simulink model "Functional_LineFollowingRobot"  (R2024a)
settings: Solver=VariableStepAuto  StartTime=0.0  StopTime=10.0  RelTol=1e-3
settings Model: Creator=pedro  LastModifiedBy=pedro

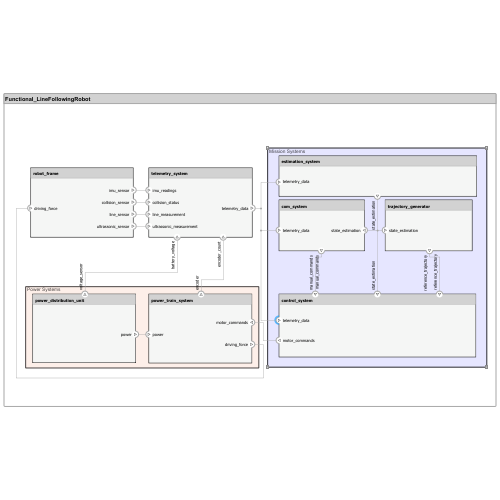
[thumbnail: Simulink's stored preview of the top-level diagram]
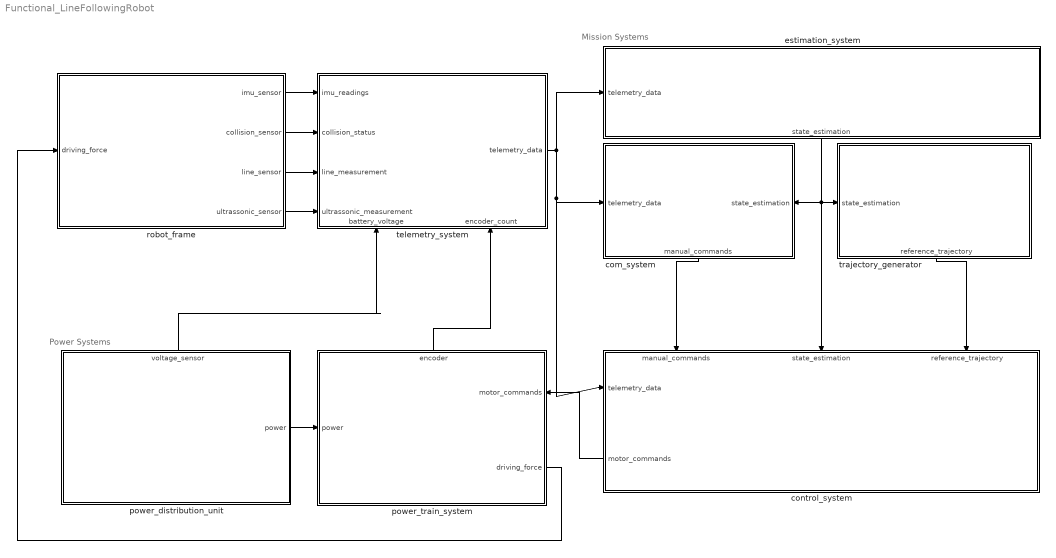
== system Functional_LineFollowingRobot ==
  note: Power Systems
  note: Mission Systems
  com_system : Subsystem
      settings: PortSchema="{\"entries\":[{\"content\":{\"headerSize\":26,\"margin\":15,\"minimumSpacing\":25,\"sides\":[{\"content\":{\"connectorIds\":[\"In2\"]},\"type\":\"ConnectorPlacement.EquallySpacedRectSide\",\"uuid\":\"4832beee-3c8d-4276-aac4-b86a684a787e\"},{\"content\":{\"connectorIds\":[\"In1\"],\"side\":\"RIGHT\"},\"type\":\"ConnectorPlacement.EquallySpacedRectSide\",\"uuid\":\"2c389b1c-5dd0-4d5d-98eb-a9eff98bcfdd\"},{\"content\":{\"side\":\"TOP\"},\"type\":\"ConnectorPlacement.EquallySpacedRectSide\",\"uuid\":\"c0c925d2-d939-46f6-a0f7-d4e3ec744eed\"},{\"content\":{\"connectorIds\":[\"Out1\"],\"side\":\"BOTTOM\"},\"type\":\"ConnectorPlacement.EquallySpacedRectSide\",\"uuid\":\"501e751b-5f5c-4d33-aa26-8cd64b6f3e74\"}]},\"type\":\"ConnectorPlacement.EquallySpacedConnector\",\"uuid\":\"424459fb-a04f-4037-ace5-d153f52e2b89\"}],\"packageUris\":[\"http://schema.mathworks.com/mf0/Connector/R2020b\"],\"version\":\"1.0\"}"
  control_system : Subsystem
      settings: PortSchema="{\"entries\":[{\"content\":{\"headerSize\":26,\"margin\":15,\"minimumSpacing\":25,\"sides\":[{\"content\":{\"connectorIds\":[\"In2\",\"Out1\"]},\"type\":\"ConnectorPlacement.EquallySpacedRectSide\",\"uuid\":\"4832beee-3c8d-4276-aac4-b86a684a787e\"},{\"content\":{\"side\":\"RIGHT\"},\"type\":\"ConnectorPlacement.EquallySpacedRectSide\",\"uuid\":\"2c389b1c-5dd0-4d5d-98eb-a9eff98bcfdd\"},{\"content\":{\"connectorIds\":[\"In1\",\"In4\",\"In3\"],\"side\":\"TOP\"},\"type\":\"ConnectorPlacement.EquallySpacedRectSide\",\"uuid\":\"c0c925d2-d939-46f6-a0f7-d4e3ec744eed\"},{\"content\":{\"side\":\"BOTTOM\"},\"type\":\"ConnectorPlacement.EquallySpacedRectSide\",\"uuid\":\"08be73b3-c42a-4f82-a3e3-56e96afeafa7\"}]},\"type\":\"ConnectorPlacement.EquallySpacedConnector\",\"uuid\":\"424459fb-a04f-4037-ace5-d153f52e2b89\"}],\"packageUris\":[\"http://schema.mathworks.com/mf0/Connector/R2020b\"],\"version\":\"1.0\"}"
  estimation_system : Subsystem
      settings: PortSchema="{\"entries\":[{\"content\":{\"headerSize\":26,\"margin\":15,\"minimumSpacing\":25,\"sides\":[{\"content\":{\"connectorIds\":[\"In1\"]},\"type\":\"ConnectorPlacement.EquallySpacedRectSide\",\"uuid\":\"4832beee-3c8d-4276-aac4-b86a684a787e\"},{\"content\":{\"side\":\"RIGHT\"},\"type\":\"ConnectorPlacement.EquallySpacedRectSide\",\"uuid\":\"2c389b1c-5dd0-4d5d-98eb-a9eff98bcfdd\"},{\"content\":{\"side\":\"TOP\"},\"type\":\"ConnectorPlacement.EquallySpacedRectSide\",\"uuid\":\"c0c925d2-d939-46f6-a0f7-d4e3ec744eed\"},{\"content\":{\"connectorIds\":[\"Out1\"],\"side\":\"BOTTOM\"},\"type\":\"ConnectorPlacement.EquallySpacedRectSide\",\"uuid\":\"d76891fa-23de-4411-a90a-4a1fbb70c268\"}]},\"type\":\"ConnectorPlacement.EquallySpacedConnector\",\"uuid\":\"424459fb-a04f-4037-ace5-d153f52e2b89\"}],\"packageUris\":[\"http://schema.mathworks.com/mf0/Connector/R2020b\"],\"version\":\"1.0\"}"
  power_distribution_unit : Subsystem
      settings: PortSchema="{\"entries\":[{\"content\":{\"headerSize\":26,\"margin\":15,\"minimumSpacing\":25,\"sides\":[{\"content\":{},\"type\":\"ConnectorPlacement.EquallySpacedRectSide\",\"uuid\":\"4832beee-3c8d-4276-aac4-b86a684a787e\"},{\"content\":{\"connectorIds\":[\"Out1\"],\"side\":\"RIGHT\"},\"type\":\"ConnectorPlacement.EquallySpacedRectSide\",\"uuid\":\"2c389b1c-5dd0-4d5d-98eb-a9eff98bcfdd\"},{\"content\":{\"connectorIds\":[\"Out2\"],\"side\":\"TOP\"},\"type\":\"ConnectorPlacement.EquallySpacedRectSide\",\"uuid\":\"c0c925d2-d939-46f6-a0f7-d4e3ec744eed\"},{\"content\":{\"side\":\"BOTTOM\"},\"type\":\"ConnectorPlacement.EquallySpacedRectSide\",\"uuid\":\"1aa9b233-1b30-4eb2-b648-626ea5c748e2\"}]},\"type\":\"ConnectorPlacement.EquallySpacedConnector\",\"uuid\":\"424459fb-a04f-4037-ace5-d153f52e2b89\"}],\"packageUris\":[\"http://schema.mathworks.com/mf0/Connector/R2020b\"],\"version\":\"1.0\"}"
  power_train_system : Subsystem
      settings: PortSchema="{\"entries\":[{\"content\":{\"headerSize\":26,\"margin\":15,\"minimumSpacing\":25,\"sides\":[{\"content\":{\"connectorIds\":[\"In2\"]},\"type\":\"ConnectorPlacement.EquallySpacedRectSide\",\"uuid\":\"4832beee-3c8d-4276-aac4-b86a684a787e\"},{\"content\":{\"connectorIds\":[\"In1\",\"Out1\"],\"side\":\"RIGHT\"},\"type\":\"ConnectorPlacement.EquallySpacedRectSide\",\"uuid\":\"2c389b1c-5dd0-4d5d-98eb-a9eff98bcfdd\"},{\"content\":{\"connectorIds\":[\"Out2\"],\"side\":\"TOP\"},\"type\":\"ConnectorPlacement.EquallySpacedRectSide\",\"uuid\":\"c0c925d2-d939-46f6-a0f7-d4e3ec744eed\"},{\"content\":{\"side\":\"BOTTOM\"},\"type\":\"ConnectorPlacement.EquallySpacedRectSide\",\"uuid\":\"cbeccc70-c914-499a-a0c2-ba0cf3f08829\"}]},\"type\":\"ConnectorPlacement.EquallySpacedConnector\",\"uuid\":\"424459fb-a04f-4037-ace5-d153f52e2b89\"}],\"packageUris\":[\"http://schema.mathworks.com/mf0/Connector/R2020b\"],\"version\":\"1.0\"}"
  robot_frame : Subsystem
      settings: PortSchema="{\"entries\":[{\"content\":{\"headerSize\":26,\"margin\":15,\"minimumSpacing\":25,\"sides\":[{\"content\":{\"connectorIds\":[\"In1\"]},\"type\":\"ConnectorPlacement.EquallySpacedRectSide\",\"uuid\":\"4832beee-3c8d-4276-aac4-b86a684a787e\"},{\"content\":{\"connectorIds\":[\"Out1\",\"Out2\",\"Out3\",\"Out4\"],\"side\":\"RIGHT\"},\"type\":\"ConnectorPlacement.EquallySpacedRectSide\",\"uuid\":\"2c389b1c-5dd0-4d5d-98eb-a9eff98bcfdd\"},{\"content\":{\"side\":\"TOP\"},\"type\":\"ConnectorPlacement.EquallySpacedRectSide\",\"uuid\":\"c0c925d2-d939-46f6-a0f7-d4e3ec744eed\"}]},\"type\":\"ConnectorPlacement.EquallySpacedConnector\",\"uuid\":\"424459fb-a04f-4037-ace5-d153f52e2b89\"}],\"packageUris\":[\"http://schema.mathworks.com/mf0/Connector/R2020b\"],\"version\":\"1.0\"}"
  telemetry_system : Subsystem
      settings: PortSchema="{\"entries\":[{\"content\":{\"headerSize\":26,\"margin\":15,\"minimumSpacing\":25,\"sides\":[{\"content\":{\"connectorIds\":[\"In1\",\"In2\",\"In3\",\"In4\"]},\"type\":\"ConnectorPlacement.EquallySpacedRectSide\",\"uuid\":\"4832beee-3c8d-4276-aac4-b86a684a787e\"},{\"content\":{\"connectorIds\":[\"Out1\"],\"side\":\"RIGHT\"},\"type\":\"ConnectorPlacement.EquallySpacedRectSide\",\"uuid\":\"2c389b1c-5dd0-4d5d-98eb-a9eff98bcfdd\"},{\"content\":{\"side\":\"TOP\"},\"type\":\"ConnectorPlacement.EquallySpacedRectSide\",\"uuid\":\"c0c925d2-d939-46f6-a0f7-d4e3ec744eed\"},{\"content\":{\"connectorIds\":[\"In5\",\"In6\"],\"side\":\"BOTTOM\"},\"type\":\"ConnectorPlacement.EquallySpacedRectSide\",\"uuid\":\"5c99a527-2db7-49a5-9f4f-18d6a8edb429\"}]},\"type\":\"ConnectorPlacement.EquallySpacedConnector\",\"uuid\":\"424459fb-a04f-4037-ace5-d153f52e2b89\"}],\"packageUris\":[\"http://schema.mathworks.com/mf0/Connector/R2020b\"],\"version\":\"1.0\"}"
  trajectory_generator : Subsystem
      settings: PortSchema="{\"entries\":[{\"content\":{\"headerSize\":26,\"margin\":15,\"minimumSpacing\":25,\"sides\":[{\"content\":{\"connectorIds\":[\"In1\"]},\"type\":\"ConnectorPlacement.EquallySpacedRectSide\",\"uuid\":\"4832beee-3c8d-4276-aac4-b86a684a787e\"},{\"content\":{\"side\":\"RIGHT\"},\"type\":\"ConnectorPlacement.EquallySpacedRectSide\",\"uuid\":\"2c389b1c-5dd0-4d5d-98eb-a9eff98bcfdd\"},{\"content\":{\"side\":\"TOP\"},\"type\":\"ConnectorPlacement.EquallySpacedRectSide\",\"uuid\":\"c0c925d2-d939-46f6-a0f7-d4e3ec744eed\"},{\"content\":{\"connectorIds\":[\"Out1\"],\"side\":\"BOTTOM\"},\"type\":\"ConnectorPlacement.EquallySpacedRectSide\",\"uuid\":\"37185e83-8287-462f-8b6c-e2b7cde56f21\"}]},\"type\":\"ConnectorPlacement.EquallySpacedConnector\",\"uuid\":\"424459fb-a04f-4037-ace5-d153f52e2b89\"}],\"packageUris\":[\"http://schema.mathworks.com/mf0/Connector/R2020b\"],\"version\":\"1.0\"}"
  wires:
  power_train_system/2(encoder) -> telemetry_system/6(encoder_count)
  power_distribution_unit/2(voltage_sensor) -> telemetry_system/5(battery_voltage)
  robot_frame/4(ultrassonic_sensor) -> telemetry_system/4(ultrassonic_measurement)
  robot_frame/3(line_sensor) -> telemetry_system/3(line_measurement)
  robot_frame/2(collision_sensor) -> telemetry_system/2(collision_status)
  telemetry_system/1(telemetry_data) -> control_system/2(telemetry_data), com_system/2(telemetry_data), estimation_system/1(telemetry_data)
  robot_frame/1(imu_sensor) -> telemetry_system/1(imu_readings)
  estimation_system/1(state_estimation) -> control_system/4(state_estimation), com_system/1(state_estimation), trajectory_generator/1(state_estimation)
  power_distribution_unit/1(power) -> power_train_system/2(power)
  control_system/1(motor_commands) -> power_train_system/1(motor_commands)
  com_system/1(manual_commands) -> control_system/1(manual_commands)
  trajectory_generator/1(reference_trajectory) -> control_system/3(reference_trajectory)
  power_train_system/1(driving_force) -> robot_frame/1(driving_force)

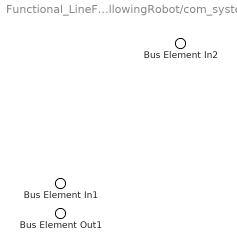
== system Functional_LineFollowingRobot/com_system ==
  Bus Element In2 : Inport  PortName=state_estimation
  Bus Element In1 : Inport  Port=2  PortName=telemetry_data
  Bus Element Out1 : Outport  PortName=manual_commands

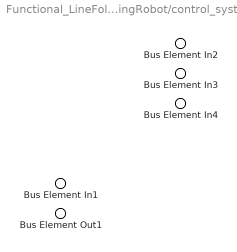
== system Functional_LineFollowingRobot/control_system ==
  Bus Element In3 : Inport  PortName=manual_commands
  Bus Element In2 : Inport  Port=2  PortName=telemetry_data
  Bus Element In4 : Inport  Port=3  PortName=reference_trajectory
  Bus Element In1 : Inport  Port=4  PortName=state_estimation
  Bus Element Out1 : Outport  PortName=motor_commands

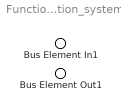
== system Functional_LineFollowingRobot/estimation_system ==
  Bus Element In1 : Inport  PortName=telemetry_data
  Bus Element Out1 : Outport  PortName=state_estimation

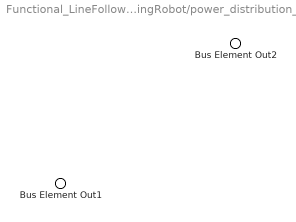
== system Functional_LineFollowingRobot/power_distribution_unit ==
  Bus Element Out2 : Outport  PortName=power
  Bus Element Out1 : Outport  Port=2  PortName=voltage_sensor

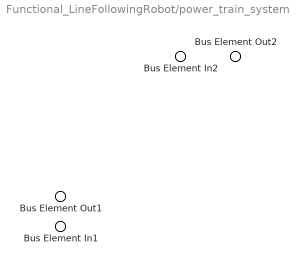
== system Functional_LineFollowingRobot/power_train_system ==
  Bus Element In2 : Inport  PortName=motor_commands
  Bus Element In1 : Inport  Port=2  PortName=power
  Bus Element Out2 : Outport  PortName=driving_force
  Bus Element Out1 : Outport  Port=2  PortName=encoder

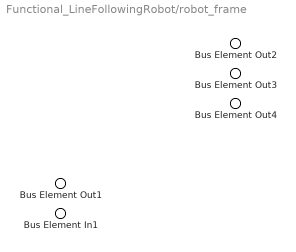
== system Functional_LineFollowingRobot/robot_frame ==
  Bus Element In1 : Inport  PortName=driving_force
  Bus Element Out4 : Outport  PortName=imu_sensor
  Bus Element Out3 : Outport  Port=2  PortName=collision_sensor
  Bus Element Out2 : Outport  Port=3  PortName=line_sensor
  Bus Element Out1 : Outport  Port=4  PortName=ultrassonic_sensor

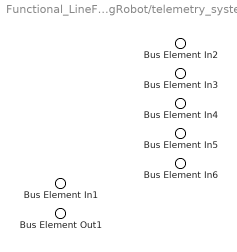
== system Functional_LineFollowingRobot/telemetry_system ==
  Bus Element In6 : Inport  PortName=imu_readings
  Bus Element In5 : Inport  Port=2  PortName=collision_status
  Bus Element In4 : Inport  Port=3  PortName=line_measurement
  Bus Element In3 : Inport  Port=4  PortName=ultrassonic_measurement
  Bus Element In2 : Inport  Port=5  PortName=battery_voltage
  Bus Element In1 : Inport  Port=6  PortName=encoder_count
  Bus Element Out1 : Outport  PortName=telemetry_data

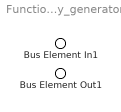
== system Functional_LineFollowingRobot/trajectory_generator ==
  Bus Element In1 : Inport  PortName=state_estimation
  Bus Element Out1 : Outport  PortName=reference_trajectory
